simulink model "GEMM_Ex3"  (R2025a)
settings: Solver=VariableStepAuto  StartTime=0.0  StopTime=10  RelTol=1e-3
undefined symbols (not defined in the file): Column, DUT, GEMM_identity, L, major, vsva1596, xcvc1702
libraries: aieDSP x1, aieUtilities x1, vmcUtilities x1
settings Model: Creator=sdegala  LastModifiedBy=robg
settings DebuggingCC: UnderspecifiedInitializationDetection=Classic  MergeDetectMultiDrivingBlocksExec=none
settings ModelReferenceCC: EnableRefExpFcnMdlSchedulingChecks=on  PropagateSignalLabelsOutOfModel=off
settings RTWCC: GPUComputeCapability=3.5

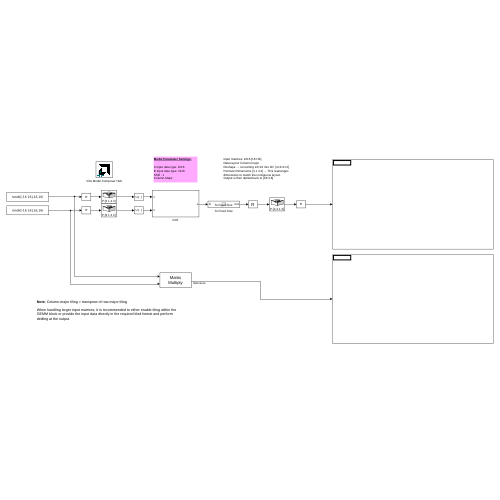
[thumbnail: Simulink's stored preview of the top-level diagram]
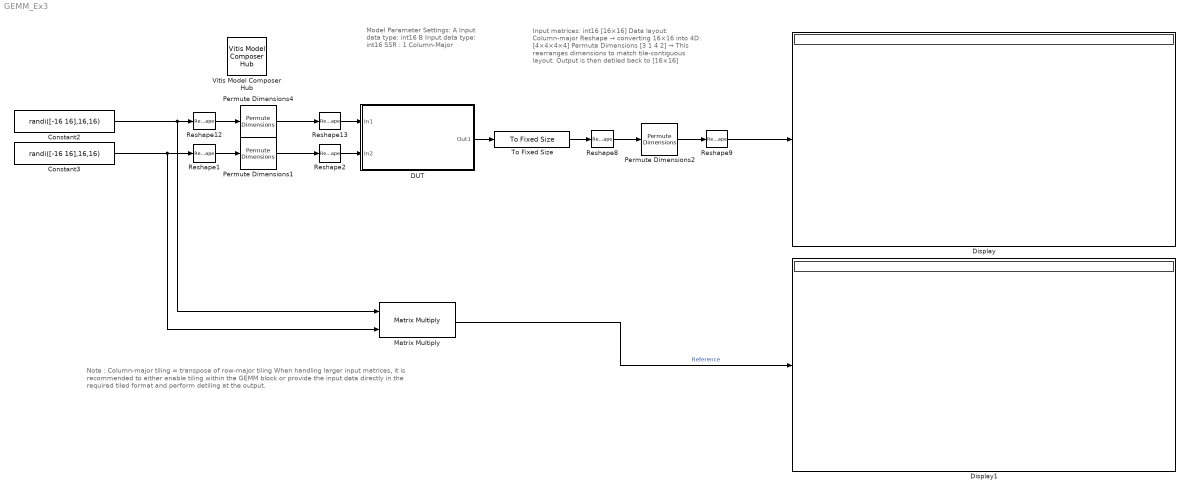
== system GEMM_Ex3 ==
  note: Note : Column-major tiling = transpose of row-major tiling
      |
      | When handling larger input matrices, it is recommended to either enable tiling within the GEMM block or provide the input data directly in the required tiled format and perform detiling at the output.
  note: Input matrices: int16 [16×16]
      | Data layout: Column-major
      | Reshape → converting 16×16 into 4D: [4×4×4×4]
      | Permute Dimensions [3 1 4 2] → This rearranges dimensions to match tile-contiguous layout.
      | Output is then detiled back to [16×16]
  note: Model Parameter Settings:
      |
      | A Input data type: int16
      | B Input data type: int16
      | SSR : 1
      | Column-Major
  Constant2 : Constant  Value=randi([-16 16],16,16)  OutDataTypeStr=int16  SampleTime=1
  Constant3 : Constant  Value=randi([-16 16],16,16)  OutDataTypeStr=int16  SampleTime=1
  DUT : Subsystem
  Display : Display
  Display1 : Display
  Matrix Multiply : Product  Multiplication=Matrix(*)  OutDataTypeStr=int16
  Permute Dimensions1 : PermuteDimensions  Order=[3 1 4 2]
  Permute Dimensions2 : PermuteDimensions  Order=[2,4,1,3]
  Permute Dimensions4 : PermuteDimensions  Order=[3 1 4 2]
  Reshape1 : Reshape  OutputDimensionality=Customize  OutputDimensions=[4,4,4,4]
  Reshape12 : Reshape  OutputDimensionality=Customize  OutputDimensions=[4,4,4,4]
  Reshape13 : Reshape
  Reshape2 : Reshape
  Reshape8 : Reshape  OutputDimensionality=Customize  OutputDimensions=[4,4,4,4]
  Reshape9 : Reshape  OutputDimensionality=Customize  OutputDimensions=[16,16]
  To Fixed Size : aieUtilities/To Fixed Size  Mode=Stop simulation when input variable-size signal is not full  OutputSize=Inherit: Same as input  CopyMethod=Buffer samples to form output  HasStatusOutput=on
  Vitis Model Composer Hub : vmcUtilities/Vitis Model Composer Hub  Tag=genX  CodeGeneration=off  SubsystemName=DUT  BlockHierPath=GEMM_identity/DUT  SubsystemType=AIENode  AIEArrayConfig=Use entire AIE array  StartColumn=1  NumberOfColumns=1  TargetDirectory=./code_bad  exportDesign=on  analyzeDesign=off  validateDesignOnHw=off  ExportType=AI Engines  IpVendor=xilinx.com  IpLibrary=hls  IpVersion=1.0  IpHWLanguage=Verilog  AieCompilerOptions={}  AieSimulatorOptions={}  CreateTestbench=on  TestbenchStackSize=10  RunRtlSim=off  RunCSim=off  RunAieSim=off  enableSimulationTimeout=on  enableGraphIterations=on  AieSimTimeout=50000  AieGraphIterations=-1  RunAieSimProfiling=off  LaunchVitisAnalyzer=off  PlotOutput=off  RunX86Sim=off  X86SimTimeout=10  GenHwImage=off  GenLibadfXo=off  GenHwValidationCode=off  PlatformType=Not Specified  HwSystemType=Baremetal  HwValidationTarget=hw  ProjDevice=xcvc1702-vsva1596-2LP-e-L  ProjDevicePart=xcvc1702-vsva1596-2LP-e-L  AIEType=AIE  SamplePeriod=-1  ClockFrequency=200  DataPathParallelism=1  xilinxfamily=versalaicore  part=xcvc1702  speed=-2LP-e-L  package=vsva1596  directory=./netlist  testbench=off  incr_netlist=off  synthesis_tool=Vivado  clock_wrapper=Clock Enables  dbl_ovrd=According to Block Masks  dcm_input_clock_period=10  sysclk_period=10  simulink_period=1  eval_field=0  IPInfoJsonString="{\"DUTSubsystemName\":\"DUT\",\"AIESubsystem\":{\"SubsystemName\":\"DUT\",\"TargetDirectory\":\"./code_bad\",\"AIEArrayConfig\":\"Use entire AIE array\",\"StartColumn\":\"0\",\"NumberOfColumns\":\"1\"},\"SubsystemTag\":\"AIENode\"}"  LogFileName=/group/xcoswmktg2/robg/scratch/CR/1263542/code_bad/model_composer.log  NThreads=4  IPConfigFile=/tmp/vmctmp-10531659881249730317/GEMM_identity_ipconfig.json
  wires:
  Matrix Multiply/1 -> Display1/1  "Reference"
  Constant2/1 -> Reshape12/1, Matrix Multiply/1
  Constant3/1 -> Reshape1/1, Matrix Multiply/2
  DUT/1(Out1) -> To Fixed Size/1
  Reshape12/1 -> Permute Dimensions4/1
  Permute Dimensions4/1 -> Reshape13/1
  Reshape13/1 -> DUT/1(In1)
  Reshape9/1 -> Display/1
  Permute Dimensions2/1 -> Reshape9/1
  Reshape8/1 -> Permute Dimensions2/1
  To Fixed Size/1 -> Reshape8/1
  Permute Dimensions1/1 -> Reshape2/1
  Reshape1/1 -> Permute Dimensions1/1
  Reshape2/1 -> DUT/2(In2)

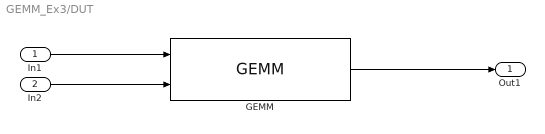
== system GEMM_Ex3/DUT ==
  In1 : Inport
  In2 : Inport  Port=2
  GEMM : aieDSP/GEMM  AIE_VARIANT=1  data_type_A=int16  data_type_B=int16  data_type_out=int16  Dim_A=16  Dim_B=16  Dim_AB=16  ssr=1  casc_length=1  InputWindowSizeA=32  InputWindowSizeB=16  A_Leading_data=Column-major(1)  B_Leading_data=Column-major(1)  Output_Leading_data=Column-major(1)  A_Tiling_data=off  B_Tiling_data=off  Output_Detiling_data=off  shift_output=0  rnd_mode=Floor  sat_mode=None  blockJsonConstraints=[]  blockJsonConstraintsInternal=[]  spec=vmc_matrix_mult.json  SerializedMaskParamNames=[]  SerializedMaskParamValues=[]  SerializedMaskParamVisibilities=[]  block_type=GEMM  SerializedMaskParamDataypes=uint|typename|typename|typename|uint|uint|uint|uint|uint|uint|uint|uint|uint|uint|uint|uint|uint|uint|uint|uint  SerializedMaskParamEnumStrArr=0|0|0|0|0|0|0|0|0|0|0|Row-major(0),Column-major(1)|Row-major(0),Column-major(1)|Row-major(0),Column-major(1)|0|0|0|0|Floor,Ceiling,Round to positive infinity,Round to negative infinity,Round symmetrical to infinity,Round symmetrical to zero,Round convergent to even,Round convergent to odd|None,Saturate,Symmetric  SerializedMaskParamEnumValArr=0|0|0|0|0|0|0|0|0|0|0|0,1|0,1|0,1|0|0|0|0|0,1,2,3,4,5,6,7|0,1,3  SerializedMaskParamVectorArr=0|0|0|0|0|0|0|0|0|0|0|0|0|0|0|0|0|0|0|0  SerializedMaskParamKeys=AIE_VARIANT|TT_DATA_A|TT_DATA_B|TT_OUT_DATA|TP_DIM_A|TP_DIM_B|TP_DIM_AB|TP_SSR|TP_CASC_LEN|TP_INPUT_WINDOW_VSIZE_A|TP_INPUT_WINDOW_VSIZE_B|TP_DIM_A_LEADING|TP_DIM_B_LEADING|TP_DIM_OUT_LEADING|TP_ADD_TILING_A|TP_ADD_TILING_B|TP_ADD_DETILING_OUT|TP_SHIFT|TP_RND|TP_SAT
  Out1 : Outport
  wires:
  In2/1 -> GEMM/2
  In1/1 -> GEMM/1
  GEMM/1 -> Out1/1
